simulink model "BSCU_Duration_tmp"  (Simulink 8.4)
settings: Solver=ode45  StartTime=0.0  StopTime=10.0  RelTol=1e-3
settings Model: Creator=bourbouh  LastModifiedBy=hbourbou  CovSFcnEnable=on
settings DataIOCC: LimitDataPoints=off  SaveFormat=StructureWithTime  SignalLoggingSaveFormat=Dataset
settings OptimizationCC: ExpressionDepthLimit=128
settings DebuggingCC: UnderspecifiedInitializationDetection=Simplified  MergeDetectMultiDrivingBlocksExec=error  SolverPrmCheckMsg=none  FcnCallInpInsideContextMsg=EnableAllAsError  FrameProcessingCompatibilityMsg=error  StateNameClashWarn=none
settings HardwareCC: ProdBitPerPointer=64  ProdLargestAtomicFloat=Float  ProdIntDivRoundTo=Zero  ProdEndianess=LittleEndian  ProdHWDeviceType=Specified
settings ModelReferenceCC: PropagateSignalLabelsOutOfModel=on
settings GRTTargetCC: CombineOutputUpdateFcns=on  GRTInterface=off

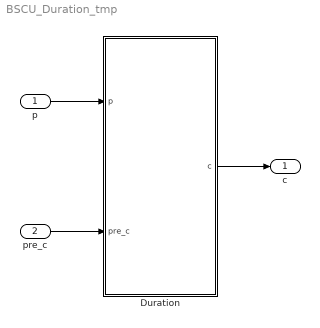
== system BSCU_Duration_tmp ==
  p : Inport
  pre_c : Inport  Port=2
  Duration : Stateflow chart  TreatAsAtomicUnit=on
      settings: PermitHierarchicalResolution=ParametersOnly
  c : Outport
  wires:
  p/1 -> Duration/1(p)
  pre_c/1 -> Duration/2(pre_c)
  Duration/1(c) -> c/1

== stateflow chart Duration ==
  (default) -> (junction 6)
  (junction 6) -> (junction 7) [order 1] : [p]
  (junction 6) -> (junction 8) [order 2] : {c = 0;}
  (junction 7) -> (junction 9) : {c = pre_c+1;}
  (junction 9) -> (junction 8)
  (junction 8) -> (junction 10)
  data: p input boolean; c output int32; pre_c input int32
